simulink model "Test"  (R2017a)
settings: Solver=VariableStepAuto  StartTime=0.0  StopTime=10.0  RelTol=1e-3
libraries: fuzblock x1
settings Model: Creator=xp  LastModifiedBy=xp

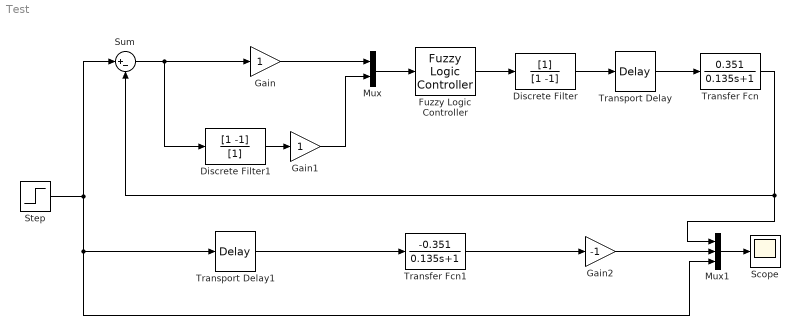
== system Test ==
  Discrete Filter : DiscreteFilter  Denominator=[1 -1]
  Discrete Filter1 : DiscreteFilter  Numerator=[1 -1]  Denominator=[1]
  Fuzzy Logic Controller : fuzblock/Fuzzy Logic  Controller  fis=[]
  Gain : Gain
  Gain1 : Gain
  Gain2 : Gain  Gain=-1
  Mux : Mux  Inputs=2
  Mux1 : Mux  Inputs=3
  Scope : Scope
  Step : Step  SampleTime=0
  Sum : Sum  Inputs=|+-
  Transfer Fcn : TransferFcn  Numerator=[0.351]  Denominator=[0.135 1]
  Transfer Fcn1 : TransferFcn  Numerator=[-0.351]  Denominator=[0.135 1]
  Transport Delay : TransportDelay
  Transport Delay1 : TransportDelay
  wires:
  Discrete Filter1/1 -> Gain1/1
  Gain/1 -> Mux/1
  Gain1/1 -> Mux/2
  Sum/1 -> Discrete Filter1/1, Gain/1
  Mux/1 -> Fuzzy Logic Controller/1
  Fuzzy Logic Controller/1 -> Discrete Filter/1
  Discrete Filter/1 -> Transport Delay/1
  Transport Delay/1 -> Transfer Fcn/1
  Mux1/1 -> Scope/1
  Gain2/1 -> Mux1/2
  Transfer Fcn1/1 -> Gain2/1
  Transport Delay1/1 -> Transfer Fcn1/1
  Step/1 -> Transport Delay1/1, Mux1/3, Sum/1
  Transfer Fcn/1 -> Sum/2, Mux1/1
